simulink model "sys_coe120"  (R2016a)
settings: Solver=VariableStepAuto  StartTime=0.0  StopTime=tend  FixedStep=Ts  RelTol=1e-3
values from neighbouring files (symbols this model uses):
  seed_nr = randi(1e4,1)    [contsid_recursiveLTV.m]
  Ts = 0.1    [contsid_TDSRIVC.m]    (also in contsid_TFCOE.m; contsid_TFFCOE.m = 0.05; contsid_TFFSRIVC.m = 0.05; contsid_TFRIVC.m)
  vare = 1e-1    (= 0.1)    [contsid_recursiveLTV.m]
settings Model: Creator=Mathieu  LastModifiedBy=arturopadilla
settings DataIOCC: LimitDataPoints=on  SaveFormat=Array  SignalLoggingSaveFormat=ModelDataLogs
settings OptimizationCC: ExpressionDepthLimit=2147483647
settings DebuggingCC: UnderspecifiedInitializationDetection=Classic  MergeDetectMultiDrivingBlocksExec=none  SolverPrmCheckMsg=warning  FcnCallInpInsideContextMsg=UseLocalSettings  AllowSymbolicDim=off  StateNameClashWarn=warning
settings HardwareCC: ProdBitPerPointer=32  ProdLargestAtomicFloat=None  ProdIntDivRoundTo=Undefined  ProdEndianess=Unspecified  ProdWordSize=32  ProdHWDeviceType=32-bit Generic
settings ModelReferenceCC: PropagateSignalLabelsOutOfModel=off
settings GRTTargetCC: CombineOutputUpdateFcns=off  GRTInterface=on
settings ConfigComp: CovModelRefEnable=Off  CovSFcnEnable=off

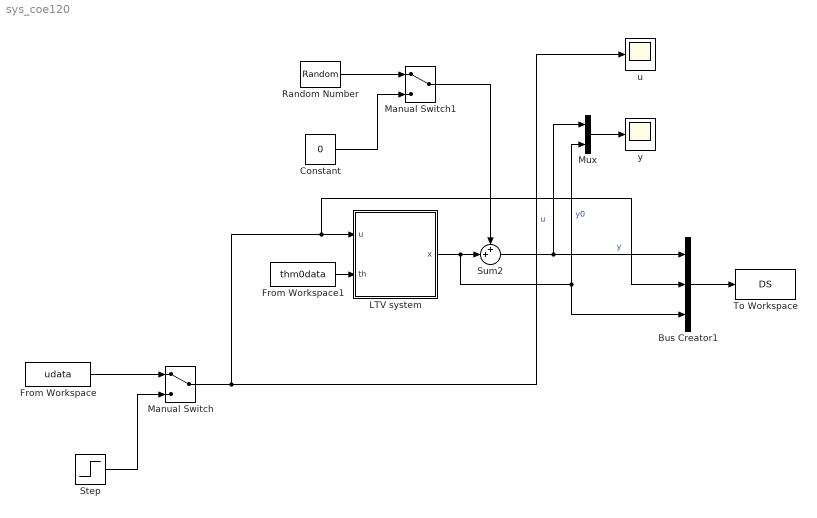
== system sys_coe120 ==
  Bus Creator1 : BusCreator  Inputs=3
  Constant : Constant  Value=0
  From Workspace : FromWorkspace  VariableName=udata  SampleTime=Ts
  From Workspace1 : FromWorkspace  VariableName=thm0data  SampleTime=Ts
  LTV system : Subsystem
  Manual Switch : ManualSwitch
  Manual Switch1 : ManualSwitch
  Mux : Mux  Inputs=2
  Random Number : RandomNumber  Variance=vare  Seed=seed_nr  SampleTime=0
  Step : Step  Time=0  SampleTime=0
  Sum2 : Sum  Inputs=++|
  To Workspace : ToWorkspace  VariableName=DS  SampleTime=Ts
  u : Scope
  y : Scope
  wires:
  Bus Creator1/1 -> To Workspace/1
  LTV system/1(x) -> Mux/2, Bus Creator1/3, Sum2/2  "y0"
  Sum2/1 -> Bus Creator1/1, Mux/1  "y"
  From Workspace/1 -> Manual Switch/1
  Manual Switch/1 -> u/1, Bus Creator1/2, LTV system/1(u)  "u"
  Step/1 -> Manual Switch/2
  Random Number/1 -> Manual Switch1/1
  Constant/1 -> Manual Switch1/2
  Manual Switch1/1 -> Sum2/1
  Mux/1 -> y/1
  From Workspace1/1 -> LTV system/2(th)

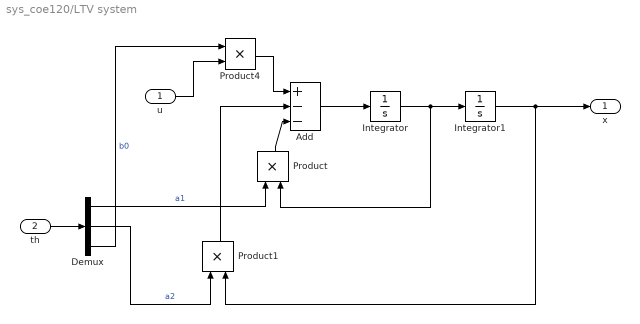
== system sys_coe120/LTV system ==
  u : Inport
  th : Inport  Port=2
  Add : Sum  Inputs=+--
  Demux : Demux  Outputs=3
  Integrator : Integrator
  Integrator1 : Integrator
  Product : Product
  Product1 : Product
  Product4 : Product  RndMeth=Zero
  x : Outport
  wires:
  Product1/1 -> Add/2
  Add/1 -> Integrator/1
  Product/1 -> Add/3
  Integrator1/1 -> Product1/2, x/1
  Integrator/1 -> Integrator1/1, Product/2
  Demux/2 -> Product1/1  "a2"
  th/1 -> Demux/1
  Demux/3 -> Product4/1  "b0"
  Demux/1 -> Product/1  "a1"
  u/1 -> Product4/2
  Product4/1 -> Add/1
